simulink model "Testmdl"  (Simulink 9.2)
settings: Solver=ode4  StartTime=0.0  StopTime=10.0  RelTol=1e-3
undefined symbols (not defined in the file or in its folder): TYP_RES_STATUS
settings Model: Creator=40005501  LastModifiedBy=40005501
settings DataIOCC: LimitDataPoints=off  SaveFormat=Dataset  SignalLoggingSaveFormat=Dataset
settings OptimizationCC: LifeSpan=auto
settings DebuggingCC: UnderspecifiedInitializationDetection=Simplified  MergeDetectMultiDrivingBlocksExec=error  FcnCallInpInsideContextMsg=error  StateNameClashWarn=none  SFUnexpectedBacktrackingDiag=error  SFNoUnconditionalDefaultTransitionDiag=error  SFExecutionAtInitializationDiag=warning
settings HardwareCC: ProdBitPerPointer=64  ProdBitPerSizeT=64  ProdBitPerPtrDiffT=64  ProdLargestAtomicFloat=Float  ProdIntDivRoundTo=Zero  ProdEndianess=LittleEndian  ProdWordSize=64  ProdHWDeviceType=Intel->x86-64 (Windows64)
settings ModelReferenceCC: PropagateSignalLabelsOutOfModel=on
settings SFSimCC: SimUseLocalCustomCode=on
settings RTWCC: RTWUseLocalCustomCode=on
settings CodeAppCC: StateflowObjectComments=off
settings GRTTargetCC: TargetLangStandard=C99 (ISO)  GeneratePreprocessorConditionals=Use local settings  CombineOutputUpdateFcns=on  GRTInterface=off
settings ConfigComp: CovMetricSettings=dwe  CovHtmlReporting=off  CovSaveCumulativeToWorkspaceVar=off  CovSaveSingleToWorkspaceVar=off  CovExternalEMLEnable=on

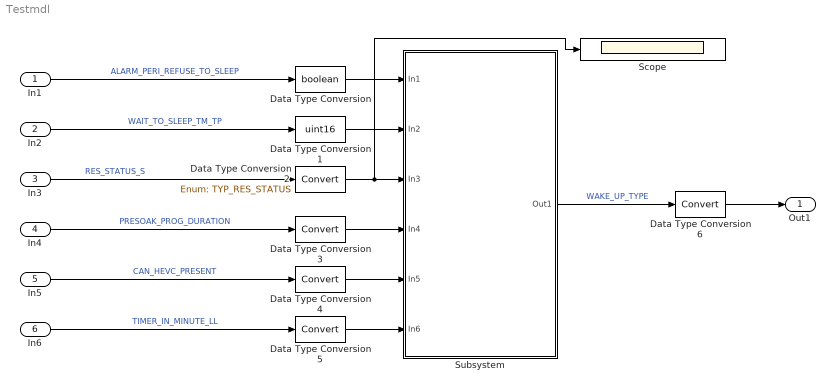
== system Testmdl ==
  In1 : Inport  OutDataTypeStr=boolean  SampleTime=0.01
  In2 : Inport  Port=2  SampleTime=0.01
  In3 : Inport  Port=3  OutDataTypeStr=Enum: TYP_RES_STATUS  SampleTime=0.01
  In4 : Inport  Port=4  OutDataTypeStr=uint8  SampleTime=0.01
  In5 : Inport  Port=5  OutDataTypeStr=boolean  SampleTime=0.01
  In6 : Inport  Port=6  OutDataTypeStr=uint16  SampleTime=0.01
  Data Type Conversion : DataTypeConversion  OutDataTypeStr=boolean
  Data Type Conversion1 : DataTypeConversion  OutDataTypeStr=uint16
  Data Type Conversion2 : DataTypeConversion  OutDataTypeStr=Enum: TYP_RES_STATUS
  Data Type Conversion{3..6} (4 alike) : DataTypeConversion
  Scope : Scope
  Subsystem : Subsystem
  Out1 : Outport  SampleTime=0.01
  wires:
  In1/1 -> Data Type Conversion/1  "ALARM_PERI_REFUSE_TO_SLEEP"
  In2/1 -> Data Type Conversion1/1  "WAIT_TO_SLEEP_TM_TP"
  In3/1 -> Data Type Conversion2/1  "RES_STATUS_S"
  In4/1 -> Data Type Conversion3/1  "PRESOAK_PROG_DURATION"
  In5/1 -> Data Type Conversion4/1  "CAN_HEVC_PRESENT"
  In6/1 -> Data Type Conversion5/1  "TIMER_IN_MINUTE_LL"
  Subsystem/1(Out1) -> Data Type Conversion6/1  "WAKE_UP_TYPE"
  Data Type Conversion/1 -> Subsystem/1(In1)
  Data Type Conversion1/1 -> Subsystem/2(In2)
  Data Type Conversion3/1 -> Subsystem/4(In4)
  Data Type Conversion4/1 -> Subsystem/5(In5)
  Data Type Conversion5/1 -> Subsystem/6(In6)
  Data Type Conversion6/1 -> Out1/1
  Data Type Conversion2/1 -> Scope/1, Subsystem/3(In3)

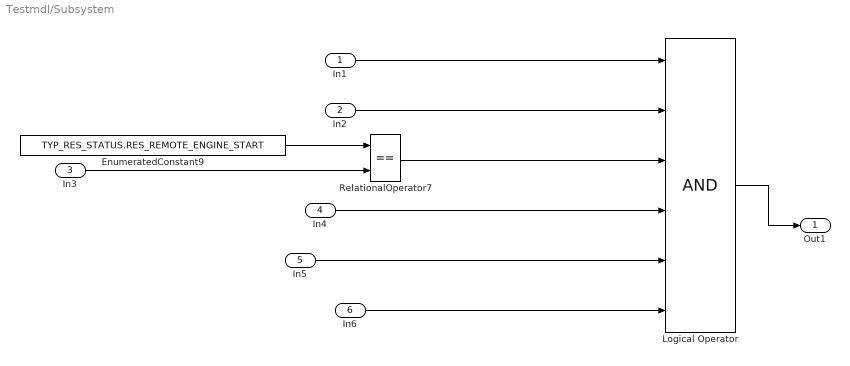
== system Testmdl/Subsystem ==
  In1 : Inport
  In2 : Inport  Port=2
  In3 : Inport  Port=3  OutDataTypeStr=Enum: TYP_RES_STATUS
  In4 : Inport  Port=4
  In5 : Inport  Port=5
  In6 : Inport  Port=6
  EnumeratedConstant9 : Constant  Value=TYP_RES_STATUS.RES_REMOTE_ENGINE_START  OutDataTypeStr=Enum: TYP_RES_STATUS  SampleTime=-1
  Logical Operator : Logic  Inputs=6  AllPortsSameDT=off  OutDataTypeStr=boolean
  RelationalOperator7 : RelationalOperator  Operator===  OutDataTypeStr=boolean  RndMeth=Nearest  InputSameDT=on
  Out1 : Outport
  wires:
  In1/1 -> Logical Operator/1
  In2/1 -> Logical Operator/2
  In4/1 -> Logical Operator/4
  In5/1 -> Logical Operator/5
  In6/1 -> Logical Operator/6
  Logical Operator/1 -> Out1/1
  EnumeratedConstant9/1 -> RelationalOperator7/1
  In3/1 -> RelationalOperator7/2
  RelationalOperator7/1 -> Logical Operator/3
